simulink model "hue_model"  (R2022a)
settings: Solver=ode45  StartTime=0.0  StopTime=20  MaxStep=0.05  RelTol=1e-3
libraries: cstblocks x2
settings Model: Creator=Valentin_Nimmervoll  LastModifiedBy=Valentin_Nimmervoll

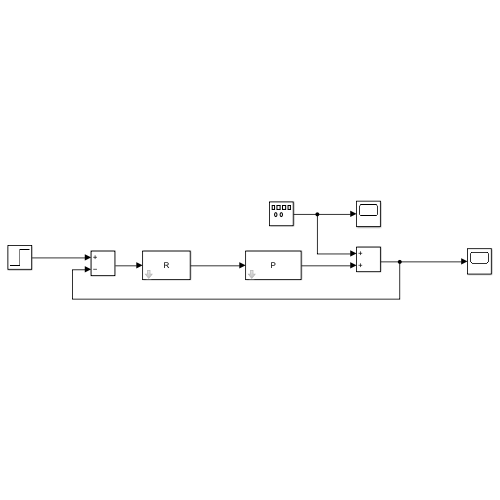
[thumbnail: Simulink's stored preview of the top-level diagram]
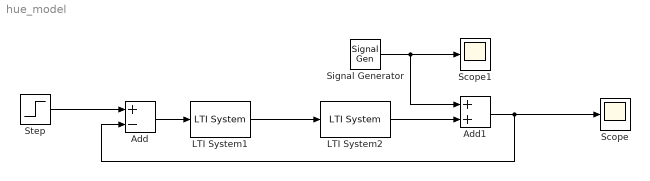
== system hue_model ==
  Add : Sum  Inputs=+-
  Add1 : Sum
  LTI System1 : cstblocks/LTI System  sys=R  IC=[]
  LTI System2 : cstblocks/LTI System  sys=P  IC=[]
  Scope : Scope
  Scope1 : Scope
  Signal Generator : SignalGenerator  Amplitude=0.7  Frequency=3  Units=rad/sec
  Step : Step  SampleTime=0
  wires:
  Step/1 -> Add/1
  Add1/1 -> Scope/1, Add/2
  Signal Generator/1 -> Add1/1, Scope1/1
  Add/1 -> LTI System1/1
  LTI System1/1 -> LTI System2/1
  LTI System2/1 -> Add1/2
